simulink model "Hsp"  (Simulink 9.2)
settings: Solver=ode23t  StartTime=0  StopTime=100  FixedStep=0.01  RelTol=1e-3  EnableMultiTasking=on
PreLoadFcn:
  |  Control;HspInit;
values from neighbouring files (symbols this model uses):
  Cep = 1.67    [HspInit.m]    (also in fuzzer_hsp.m; hsp_data.mat)
  Cev = 50.0    (= 50)    [HspInit.m]    (also in fuzzer_hsp.m; hsp_data.mat)
  Cla = 19.23    [HspInit.m]    (also in fuzzer_hsp.m; hsp_data.mat)
  Cpa = 0.76    [HspInit.m]    (also in fuzzer_hsp.m; hsp_data.mat)
  Cpp = 5.80    (= 5.8)    [HspInit.m]    (also in fuzzer_hsp.m; hsp_data.mat)
  Cpv = 25.37    [HspInit.m]    (also in fuzzer_hsp.m; hsp_data.mat)
  Cra = 31.25    [HspInit.m]    (also in fuzzer_hsp.m; hsp_data.mat)
  Csa = 0.28    [HspInit.m]    (also in fuzzer_hsp.m; hsp_data.mat)
  Csp = 2.05    [HspInit.m]    (also in fuzzer_hsp.m; hsp_data.mat)
  Csv = 61.11    [HspInit.m]    (also in fuzzer_hsp.m; hsp_data.mat)
  Dx = [  2     2     2     2    5      5        2   0.2 ]'    [Control.m]    (also in fuzzer_hsp.m; hsp_control.mat = [2 2 2 2 5 5 2 0.2])
  fcs0 = 25    [Control.m]    (also in fuzzer_hsp.m; hsp_control.mat)
  fes0 = 16.11    [Control.m]    (also in fuzzer_hsp.m; hsp_control.mat)
  fes1 = 2.10    (= 2.1)    [Control.m]    (also in fuzzer_hsp.m; hsp_control.mat)
  fesmin = 2.66    [Control.m]    (also in fuzzer_hsp.m; hsp_control.mat)
  fev0 = 3.2    [Control.m]    (also in fuzzer_hsp.m; hsp_control.mat)
  fev1 = 6.3    [Control.m]    (also in fuzzer_hsp.m; hsp_control.mat)
  fmax = 47.78    [Control.m]    (also in fuzzer_hsp.m; hsp_control.mat)
  fmin = 2.52    [Control.m]    (also in fuzzer_hsp.m; hsp_control.mat)
  Gx = [0.475 0.282  0.695 0.53 -265.4 -132.5  -0.13 0.09]'    [Control.m]    (also in fuzzer_hsp.m; hsp_control.mat = [0.475 0.282 0.695 0.53 -265.4 -132.5 -0.13 0.09])
  initx = [2.392 1.412  2.49  0.78 1435.4  1537    0.58   0]'    [Control.m]    (also in fuzzer_hsp.m; hsp_control.mat = [2.392 1.412 2.49 0.78 1435.4 1537 0.58 0])
  ka = 11.758    [Control.m]    (also in fuzzer_hsp.m; hsp_control.mat)
  KElv = 0.014    [HspInit.m]    (also in fuzzer_hsp.m; hsp_data.mat)
  KErv = 0.011    [HspInit.m]    (also in fuzzer_hsp.m; hsp_data.mat)
  kes = 0.0675    [Control.m]    (also in fuzzer_hsp.m; hsp_control.mat)
  kev = 7.06    [Control.m]    (also in fuzzer_hsp.m; hsp_control.mat)
  KRlv = 3.75e-4    (= 0.000375)    [HspInit.m]    (also in fuzzer_hsp.m; hsp_data.mat)
  KRrv = 1.4e-3    (= 0.0014)    [HspInit.m]    (also in fuzzer_hsp.m; hsp_data.mat)
  ksys = 0.075    [HspInit.m]    (also in fuzzer_hsp.m; hsp_data.mat)
  Lpa = 0.18e-3    (= 0.00018)    [HspInit.m]    (also in fuzzer_hsp.m; hsp_data.mat)
  Lsa = 0.22e-3    (= 0.00022)    [HspInit.m]    (also in fuzzer_hsp.m; hsp_data.mat)
  P0lv = 1.5    [HspInit.m]    (also in fuzzer_hsp.m; hsp_data.mat)
  P0rv = 1.5    [HspInit.m]    (also in fuzzer_hsp.m; hsp_data.mat)
  Pn = 92    [Control.m]    (also in fuzzer_hsp.m; hsp_control.mat)
  Rev = 0.016    [HspInit.m]    (also in fuzzer_hsp.m; hsp_data.mat = 0.0336)
  Rla = 25e-3    (= 0.025)    [HspInit.m]    (also in fuzzer_hsp.m; hsp_data.mat)
  Rpa = 0.023    [HspInit.m]    (also in fuzzer_hsp.m; hsp_data.mat = 0.0483)
  Rpp = 0.0894    [HspInit.m]    (also in fuzzer_hsp.m; hsp_data.mat = 0.18774)
  Rpv = 0.0056    [HspInit.m]    (also in fuzzer_hsp.m; hsp_data.mat = 0.01176)
  Rra = 2.5e-3    (= 0.0025)    [HspInit.m]    (also in fuzzer_hsp.m; hsp_data.mat)
  Rsa = 0.06    [HspInit.m]    (also in fuzzer_hsp.m; hsp_data.mat = 0.126)
  Rsv = 0.038    [HspInit.m]    (also in fuzzer_hsp.m; hsp_data.mat = 0.0798)
  toup = 2.076    [Control.m]    (also in fuzzer_hsp.m; hsp_control.mat)
  toux = [  8     8     6     6    20     20       2   1.5 ]'    [Control.m]    (also in fuzzer_hsp.m; hsp_control.mat = [8 8 6 6 20 20 2 1.5])
  touz = 6.37    [Control.m]    (also in fuzzer_hsp.m; hsp_control.mat)
  Tsys0 = 0.5    [HspInit.m]    (also in fuzzer_hsp.m; hsp_data.mat)
  Vt = 5300    [HspInit.m]    (also in fuzzer_hsp.m; hsp_data.mat)
  Vuep = 336.6    [HspInit.m]    (also in fuzzer_hsp.m; hsp_data.mat)
  Vula = 25    [HspInit.m]    (also in fuzzer_hsp.m; hsp_data.mat)
  Vulv = 16.77    [HspInit.m]    (also in fuzzer_hsp.m; hsp_data.mat)
  Vupa = 0    [HspInit.m]    (also in fuzzer_hsp.m; hsp_data.mat)
  Vupp = 123    [HspInit.m]    (also in fuzzer_hsp.m; hsp_data.mat)
  Vupv = 120    [HspInit.m]    (also in fuzzer_hsp.m; hsp_data.mat)
  Vura = 25    [HspInit.m]    (also in fuzzer_hsp.m; hsp_data.mat)
  Vurv = 40.8    [HspInit.m]    (also in fuzzer_hsp.m; hsp_data.mat)
  Vusa = 0    [HspInit.m]    (also in fuzzer_hsp.m; hsp_data.mat)
  Vusp = 274.4    [HspInit.m]    (also in fuzzer_hsp.m; hsp_data.mat)
libraries: simulink x1
CloseFcn:
  | close(findobj(allchild(0),'flat','name','HSP Data Center'));close(findobj(allchild(0),'flat','name','HSP Control Center'))
settings Model: LogicAnalyzerSignalOrdering=c852cb86-1eca-462a-854a-a1c1cbc38954,16da165e-0cbb-4ec2-850a-f71467b3fe42,a6bbb533-7671-4afb-b402-0dcba4b3517f,2284c783-9622-40c3-a6e2-0c1aa7a75d76,7db0d47d-b44d-44ed-95d3-6c2fe47389a0,23f4d4c7-257a-4786-8ae9-d827889f7a35,431a2e10-1d5e-4ec4-bfdf-46f0ec12685f,2c1b38cc-318d-4d33-94a3-ee406883b660,ecc0bcf3-2ebb-404e-884d-df489637ffdc,a0b08e82-c84b-4593-bb1c-8e64f6c8e753,b59d5f8b-8f7e-4c99-855a-97b147fb0b9b,22f6e1f3-01a7-4b2a-becd-6a35e85c0c19,b19c4093-726d-4120-89b8-8ec6b172c3ea,cea4f0ff-484e-4aeb-9f42-7c30204549fe,be0e3e8a-096d-45ad-a129-bf43744257a6  Creator=josie  LastModifiedBy=josie  ExtModeTrigMode=oneshot  ExtModeArmWhenConnect=off
settings Model: LogicAnalyzerGraphicalSettings=|
  | {
  |   "cursors" : {
  |     "activeCursor" : 0,
  |     "lockedCursors" : [
  | 
  |     ],
  |     "startingCursor" : 0,
  |     "times" : [
  |       0
  |     ]
  |   },
  |   "global" : {
  |   },
  |   "panels" : [
  |     {
  |       "height" : 100,
  |       "startingTrace" : 0,
  |       "traces" : [
  |         {
  |           "signalId" : "2284c783-9622-40c3-a6e2-0c1aa7a75d76",
  |           "type" : "wave"
  |         },
  |         {
  |           "signalId" : "2c1b38cc-318d-4d33-94a3-ee406883b660",
  |           "type" : "wave"
  |         },
  |         {
  |           "signalId" : "ecc0bcf3-2ebb-404e-884d-df489637ffdc",
  |           "type" : "wave"
  |         },
  |         {
  |           "signalId" : "a0b08e82-c84b-4593-bb1c-8e64f6c8e753",
  |           "type" : "wave"
  |         },
  |         {
  |           "signalId" : "b59d5f8b-8f7e-4c99-855a-97b147fb0b9b",
  |           "type" : "wave"
  |         },
  |         {
  |           "signalId" : "22f6e1f3-01a7-4b2a-becd-6a35e85c0c19",
  |           "type" : "wave"
  |         },
  |         {
  |           "signalId" : "b19c4093-726d-4120-89b8-8ec6b172c3ea",
  |           "type" : "wave"
  |         },
  |         {
  |           "signalId" : "cea4f0ff-484e-4aeb-9f42-7c30204549fe",
  |           "type" : "wave"
  |         },
  |         {
  |           "signalId" : "be0e3e8a-096d-45ad-a129-bf43744257a6",
  |           "type" : "wave"
  |         },
  |         {
  |           "signalId" : "b284ce3d-31c8-45a4-96bc-bbba7044bc82",
  |           "type" : "wave"
  |         }
  |       ],
  |       "yOffset" : 0
  |     }
  |   ],
  |   "timeAxis" : {
  |     "pixelsPerSecond" : 17.79
  |   },
  |   "trigger" : {
  |     "enabled" : false,
  |     "mode" : "once",
  |     "samples" : 200,
  |     "signals" : {
  |     },
  |     "stages" : [
  |       {
  |         "conditions" : [
  | 
  |         ],
  |         "operator" : "AND"
  |       }
  |     ]
  |   }
  | }
settings DataIOCC: InitialState=xFinal  LimitDataPoints=off  SaveFinalState=on  SignalLoggingSaveFormat=Dataset  SaveOutput=off
settings OptimizationCC: BlockReduction=off  BooleanDataType=off  LifeSpan=auto
settings DebuggingCC: SaveWithParameterizedLinksMsg=none  SignalResolutionControl=TryResolveAllWithWarning  MultiTaskDSMMsg=warning  MultiTaskCondExecSysMsg=none  FcnCallInpInsideContextMsg=error  StateNameClashWarn=none  SFUnexpectedBacktrackingDiag=error  SFNoUnconditionalDefaultTransitionDiag=error  SFExecutionAtInitializationDiag=warning
settings HardwareCC: ProdBitPerPointer=64  ProdBitPerSizeT=64  ProdBitPerPtrDiffT=64  ProdLargestAtomicFloat=Float  ProdIntDivRoundTo=Zero  ProdEndianess=LittleEndian  ProdWordSize=64  ProdHWDeviceType=Intel->x86-64 (Windows64)  TargetUnknown=on
settings SFSimCC: SimUseLocalCustomCode=on
settings RTWCC: RTWUseLocalCustomCode=on
settings CodeAppCC: StateflowObjectComments=off
settings GRTTargetCC: TargetLangStandard=C99 (ISO)  GeneratePreprocessorConditionals=Use local settings
settings ConfigComp: CovMetricSettings=dwe  CovSaveCumulativeToWorkspaceVar=off  CovSaveSingleToWorkspaceVar=off  CovExternalEMLEnable=on

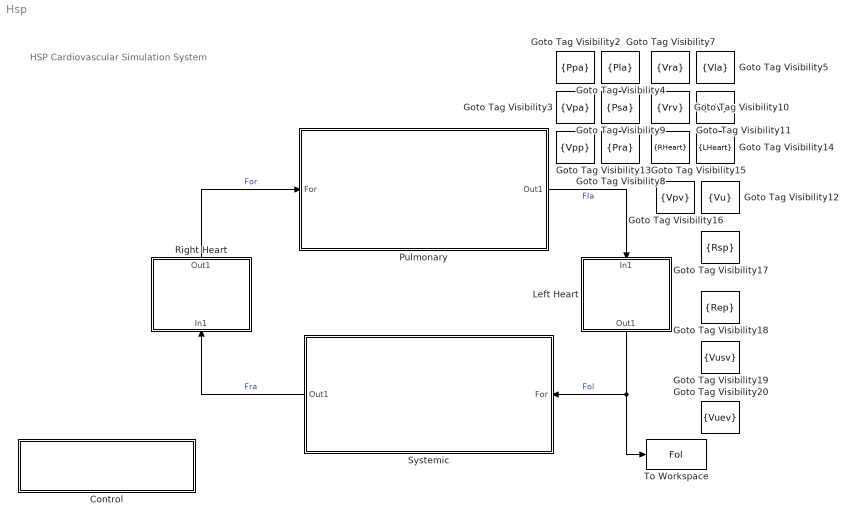
== system Hsp ==
  note: HSP
      | Cardiovascular Simulation System
  Control : Subsystem
      mask Display: disp('ANALYSIS & CONTROL SYSTEM')
  Goto Tag Visibility10 : GotoTagVisibility  GotoTag=Vrv
  Goto Tag Visibility11 : GotoTagVisibility  GotoTag=Vlv
  Goto Tag Visibility12 : GotoTagVisibility  GotoTag=Vu
  Goto Tag Visibility13 : GotoTagVisibility  GotoTag=Vpp
  Goto Tag Visibility14 : GotoTagVisibility  GotoTag=LHeart
  Goto Tag Visibility15 : GotoTagVisibility  GotoTag=RHeart
  Goto Tag Visibility16 : GotoTagVisibility  GotoTag=Vpv
  Goto Tag Visibility17 : GotoTagVisibility  GotoTag=Rsp
  Goto Tag Visibility18 : GotoTagVisibility  GotoTag=Rep
  Goto Tag Visibility19 : GotoTagVisibility  GotoTag=Vusv
  Goto Tag Visibility2 : GotoTagVisibility  GotoTag=Ppa
  Goto Tag Visibility20 : GotoTagVisibility  GotoTag=Vuev
  Goto Tag Visibility3 : GotoTagVisibility  GotoTag=Vpa
  Goto Tag Visibility4 : GotoTagVisibility  GotoTag=Pla
  Goto Tag Visibility5 : GotoTagVisibility  GotoTag=Vla
  Goto Tag Visibility7 : GotoTagVisibility  GotoTag=Vra
  Goto Tag Visibility8 : GotoTagVisibility  GotoTag=Pra
  Goto Tag Visibility9 : GotoTagVisibility  GotoTag=Psa
  Left Heart : Subsystem
      mask Display: disp('LEFT HEART')
  Pulmonary : Subsystem
      mask Display: disp('PULMONARY CIRCULATORY SYSTEM')
  Right Heart : Subsystem
      mask Display: disp('RIGHT HEART')
  Systemic : Subsystem
      mask Display: disp('SYSTEMIC CIRULATORY SYSTEM')
  To Workspace : ToWorkspace  VariableName=Fol  SampleTime=-1
  wires:
  Pulmonary/1(Out1) -> Left Heart/1(In1)  "Fla"
  Systemic/1(Out1) -> Right Heart/1(In1)  "Fra"
  Left Heart/1(Out1) -> Systemic/1(For), To Workspace/1  "Fol"
  Right Heart/1(Out1) -> Pulmonary/1(For)  "For"

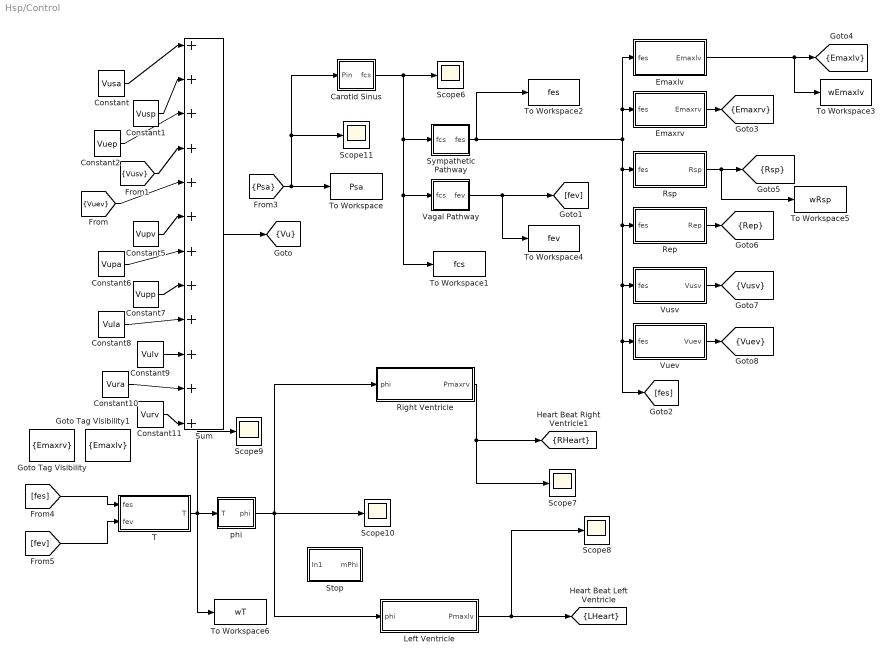
== system Hsp/Control ==
  Carotid Sinus : Subsystem
  Constant : Constant  Value=Vusa
  Constant1 : Constant  Value=Vusp
  Constant10 : Constant  Value=Vura
  Constant11 : Constant  Value=Vurv
  Constant2 : Constant  Value=Vuep
  Constant5 : Constant  Value=Vupv
  Constant6 : Constant  Value=Vupa
  Constant7 : Constant  Value=Vupp
  Constant8 : Constant  Value=Vula
  Constant9 : Constant  Value=Vulv
  Emaxlv : Subsystem
  Emaxrv : Subsystem
  Goto Tag Visibility : GotoTagVisibility  GotoTag=Emaxrv
  Goto Tag Visibility1 : GotoTagVisibility  GotoTag=Emaxlv
  Left Ventricle : Subsystem
  Rep : Subsystem
  Right Ventricle : Subsystem
  Rsp : Subsystem
  Scope{6..11} (6 alike) : Scope
  Stop : Subsystem
  Sum : Sum  Inputs=|++++++++++++  SaturateOnIntegerOverflow=on  InputSameDT=on  OutDataTypeStr=Inherit: Same as first input
  Sympathetic Pathway : Subsystem
  T : Subsystem
  To Workspace : ToWorkspace  VariableName=Psa  SampleTime=-1
  To Workspace1 : ToWorkspace  VariableName=fcs  SampleTime=-1
  To Workspace2 : ToWorkspace  VariableName=fes  SampleTime=-1
  To Workspace3 : ToWorkspace  VariableName=wEmaxlv  SampleTime=-1
  To Workspace4 : ToWorkspace  VariableName=fev  SampleTime=-1
  To Workspace5 : ToWorkspace  VariableName=wRsp  SampleTime=-1
  To Workspace6 : ToWorkspace  VariableName=wT  SampleTime=-1
  Vagal Pathway : Subsystem
  Vuev : Subsystem
  Vusv : Subsystem
  phi : Subsystem
  tag scope: Emaxlv=scoped, Emaxrv=scoped, LHeart=scoped, RHeart=scoped, Rep=scoped, Rsp=scoped, Vu=scoped, Vuev=scoped, Vusv=scoped
  wires:
  Sum/1 -> [Vu]
  Constant/1 -> Sum/1
  Constant2/1 -> Sum/3
  Constant1/1 -> Sum/2
  [Vusv] -> Sum/4
  [Vuev] -> Sum/5
  Constant5/1 -> Sum/6
  Constant6/1 -> Sum/7
  Constant7/1 -> Sum/8
  Constant8/1 -> Sum/9
  Constant9/1 -> Sum/10
  Constant10/1 -> Sum/11
  Constant11/1 -> Sum/12
  Carotid Sinus/1(fcs) -> Scope6/1, Sympathetic Pathway/1(fcs), Vagal Pathway/1(fcs), To Workspace1/1
  [fes] -> T/1(fes)
  [fev] -> T/2(fev)
  phi/1(phi) -> Scope10/1, Right Ventricle/1(phi), Left Ventricle/1(phi)
  Right Ventricle/1(Pmaxrv) -> [RHeart], Scope7/1
  Left Ventricle/1(Pmaxlv) -> [LHeart], Scope8/1
  Sympathetic Pathway/1(fes) -> Emaxlv/1(fes), Emaxrv/1(fes), Rsp/1(fes), Rep/1(fes), Vusv/1(fes), Vuev/1(fes), [fes], To Workspace2/1
  Emaxrv/1(Emaxrv) -> [Emaxrv]
  Rep/1(Rep) -> [Rep]
  Vusv/1(Vusv) -> [Vusv]
  Vuev/1(Vuev) -> [Vuev]
  Vagal Pathway/1(fev) -> [fev], To Workspace4/1
  Rsp/1(Rsp) -> [Rsp], To Workspace5/1
  [Psa] -> To Workspace/1, Scope11/1, Carotid Sinus/1(Pin)
  T/1(T) -> Scope9/1, To Workspace6/1, phi/1(T)
  Emaxlv/1(Emaxlv) -> [Emaxlv], To Workspace3/1

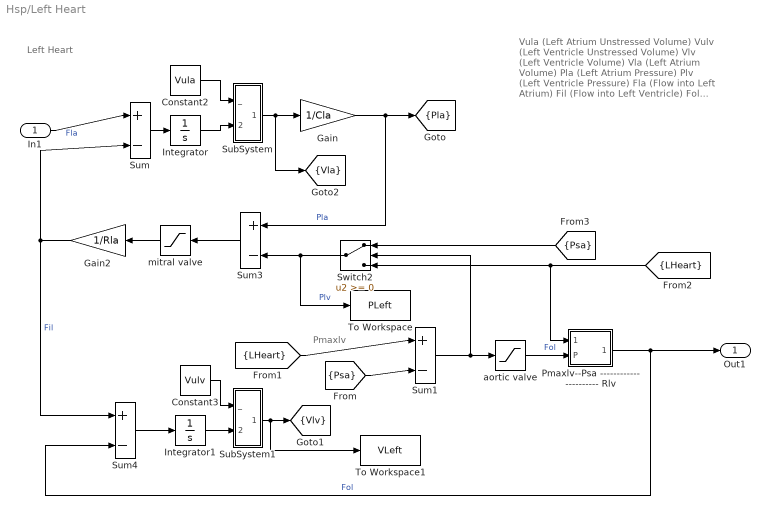
== system Hsp/Left Heart ==
  note: Left Heart
  note: Vula (Left Atrium Unstressed Volume)
      | Vulv (Left Ventricle Unstressed Volume)
      | Vlv (Left Ventricle Volume)
      | Vla (Left Atrium Volume)
      | Pla (Left Atrium Pressure)
      | Plv (Left Ventricle Pressure)
      | Fla (Flow into Left Atrium)
      | Fil (Flow into Left Ventricle)
      | Fol (Flow out of Left Ventricle)
      | LHeart (Left Ventricle Function)
  note: Pmaxlv
  In1 : Inport
  Constant2 : Constant  Value=Vula
  Constant3 : Constant  Value=Vulv
  Gain : Gain  Gain=1/Cla  SaturateOnIntegerOverflow=on  OutDataTypeStr=Inherit: Same as input  ParamDataTypeStr=Inherit: Same as input
  Gain2 : Gain  Gain=1/Rla  SaturateOnIntegerOverflow=on  OutDataTypeStr=Inherit: Same as input  ParamDataTypeStr=Inherit: Same as input
  Integrator : Integrator
  Integrator1 : Integrator
  Pmaxlv--Psa ---------------------- Rlv : Subsystem
  SubSystem : Subsystem
  SubSystem1 : Subsystem
  Sum : Sum  Inputs=|+-  SaturateOnIntegerOverflow=on  InputSameDT=on  OutDataTypeStr=Inherit: Same as first input
  Sum1 : Sum  Inputs=|+-  SaturateOnIntegerOverflow=on  InputSameDT=on  OutDataTypeStr=Inherit: Same as first input
  Sum3 : Sum  Inputs=+-  SaturateOnIntegerOverflow=on  InputSameDT=on  OutDataTypeStr=Inherit: Same as first input
  Sum4 : Sum  Inputs=+-  SaturateOnIntegerOverflow=on  InputSameDT=on  OutDataTypeStr=Inherit: Same as first input
  Switch2 : Switch  SaturateOnIntegerOverflow=on  InputSameDT=on
  To Workspace : ToWorkspace  VariableName=PLeft  SampleTime=-1
  To Workspace1 : ToWorkspace  VariableName=VLeft  SampleTime=-1
  aortic valve : Saturate  UpperLimit=inf  LowerLimit=0
  mitral valve : Saturate  UpperLimit=inf  LowerLimit=0
  Out1 : Outport
  tag scope: Pla=scoped, Vla=scoped, Vlv=scoped
  wires:
  In1/1 -> Sum/1  "Fla"
  Sum/1 -> Integrator/1
  [Psa] -> Sum1/2
  Gain/1 -> [Pla], Sum3/1  "Pla"
  Sum4/1 -> Integrator1/1
  Gain2/1 -> Sum/2, Sum4/1  "Fil"
  Pmaxlv--Psa ---------------------- Rlv/1(Flow) -> Out1/1, Sum4/2  "Fol"
  Constant2/1 -> SubSystem/1(_)
  Constant3/1 -> SubSystem1/1(_)
  SubSystem/1(Out) -> Gain/1, [Vla]
  [LHeart] -> Sum1/1
  Sum1/1 -> aortic valve/1, Switch2/2
  [Psa] -> Switch2/1
  mitral valve/1 -> Gain2/1
  [LHeart] -> Switch2/3, Pmaxlv--Psa ---------------------- Rlv/1(Pmax)
  aortic valve/1 -> Pmaxlv--Psa ---------------------- Rlv/2(P)  "Fol"
  Switch2/1 -> Sum3/2, To Workspace/1  "Plv"
  SubSystem1/1(Out) -> [Vlv], To Workspace1/1
  Integrator1/1 -> SubSystem1/2(+)
  Sum3/1 -> mitral valve/1
  Integrator/1 -> SubSystem/2(+)

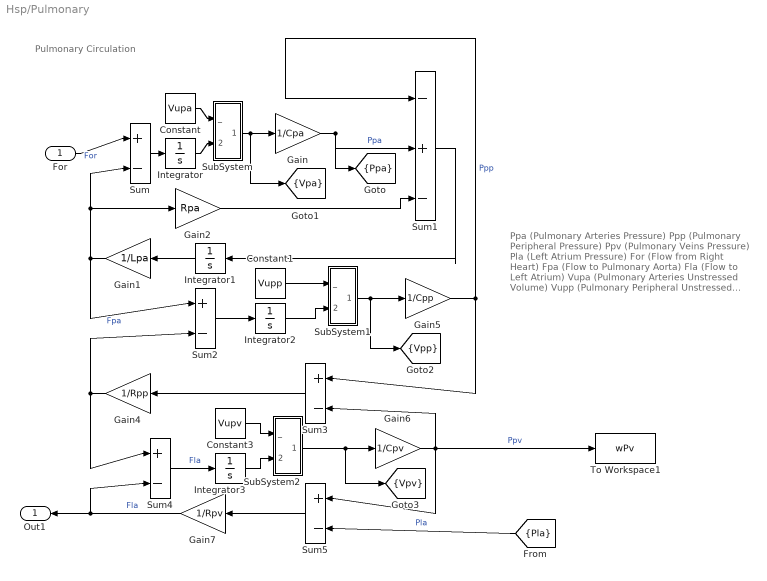
== system Hsp/Pulmonary ==
  note: Ppa (Pulmonary Arteries Pressure)
      | Ppp (Pulmonary Peripheral Pressure)
      | Ppv (Pulmonary Veins Pressure)
      | Pla (Left Atrium Pressure)
      | For (Flow from Right Heart)
      | Fpa (Flow to Pulmonary Aorta)
      | Fla (Flow to Left Atrium)
      | Vupa (Pulmonary Arteries Unstressed Volume)
      | Vupp (Pulmonary Peripheral Unstressed Volume)
      | Vupv (Pulmonary Veins Unstressed Volume)
  note: Pulmonary Circulation
  For : Inport
  Constant : Constant  Value=Vupa
  Constant1 : Constant  Value=Vupp
  Constant3 : Constant  Value=Vupv
  Gain : Gain  Gain=1/Cpa  SaturateOnIntegerOverflow=on  OutDataTypeStr=Inherit: Same as input  ParamDataTypeStr=Inherit: Same as input
  Gain1 : Gain  Gain=1/Lpa  SaturateOnIntegerOverflow=on  OutDataTypeStr=Inherit: Same as input  ParamDataTypeStr=Inherit: Same as input
  Gain2 : Gain  Gain=Rpa  SaturateOnIntegerOverflow=on  OutDataTypeStr=Inherit: Same as input  ParamDataTypeStr=Inherit: Same as input
  Gain4 : Gain  Gain=1/Rpp  SaturateOnIntegerOverflow=on  OutDataTypeStr=Inherit: Same as input  ParamDataTypeStr=Inherit: Same as input
  Gain5 : Gain  Gain=1/Cpp  SaturateOnIntegerOverflow=on  OutDataTypeStr=Inherit: Same as input  ParamDataTypeStr=Inherit: Same as input
  Gain6 : Gain  Gain=1/Cpv  SaturateOnIntegerOverflow=on  OutDataTypeStr=Inherit: Same as input  ParamDataTypeStr=Inherit: Same as input
  Gain7 : Gain  Gain=1/Rpv  SaturateOnIntegerOverflow=on  OutDataTypeStr=Inherit: Same as input  ParamDataTypeStr=Inherit: Same as input
  Integrator : Integrator  InitialCondition=100
  Integrator1 : Integrator
  Integrator2 : Integrator  InitialCondition=100
  Integrator3 : Integrator
  SubSystem : Subsystem
  SubSystem1 : Subsystem
  SubSystem2 : Subsystem
  Sum{,2..5} (5 alike) : Sum  Inputs=|+-  SaturateOnIntegerOverflow=on  InputSameDT=on  OutDataTypeStr=Inherit: Same as first input
  Sum1 : Sum  Inputs=|-+-  SaturateOnIntegerOverflow=on  InputSameDT=on  OutDataTypeStr=Inherit: Same as first input
  To Workspace1 : ToWorkspace  VariableName=wPv  SampleTime=-1
  Out1 : Outport
  tag scope: Ppa=scoped, Vpa=scoped, Vpp=scoped, Vpv=scoped
  wires:
  For/1 -> Sum/1  "For"
  Sum/1 -> Integrator/1
  Integrator1/1 -> Gain1/1
  Sum1/1 -> Integrator1/1
  Gain2/1 -> Sum1/3
  Gain1/1 -> Sum/2, Gain2/1, Sum2/1  "Fpa"
  Sum2/1 -> Integrator2/1
  Gain5/1 -> Sum1/1, Sum3/1  "Ppp"
  Sum3/1 -> Gain4/1
  Gain4/1 -> Sum2/2, Sum4/1
  Sum5/1 -> Gain7/1
  Gain6/1 -> Sum3/2, Sum5/1, To Workspace1/1  "Ppv"
  [Pla] -> Sum5/2  "Pla"
  Sum4/1 -> Integrator3/1  "Fla"
  Gain/1 -> Sum1/2, [Ppa]  "Ppa"
  SubSystem/1(Out) -> Gain/1, [Vpa]
  SubSystem1/1(Out) -> Gain5/1, [Vpp]
  SubSystem2/1(Out) -> Gain6/1, [Vpv]
  Integrator/1 -> SubSystem/2(+)
  Constant/1 -> SubSystem/1(_)
  Constant1/1 -> SubSystem1/1(_)
  Integrator2/1 -> SubSystem1/2(+)
  Integrator3/1 -> SubSystem2/2(+)
  Gain7/1 -> Sum4/2, Out1/1  "Fla"
  Constant3/1 -> SubSystem2/1(_)

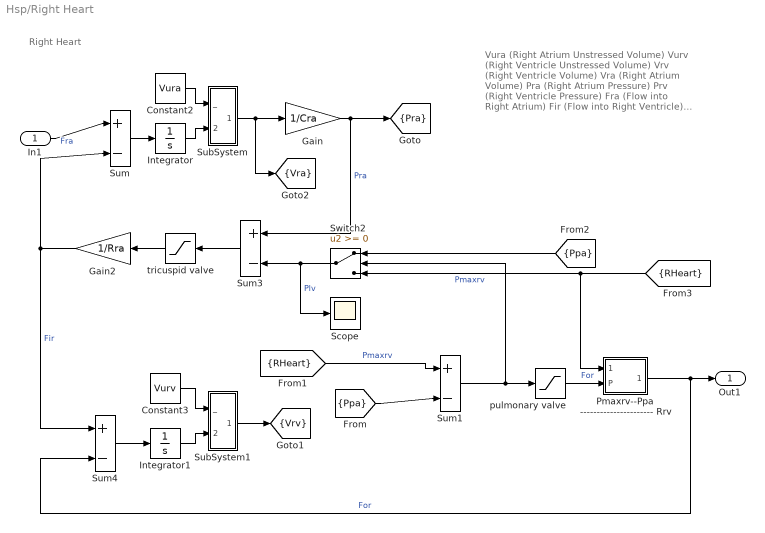
== system Hsp/Right Heart ==
  note: Right Heart
  note: Vura (Right Atrium Unstressed Volume)
      | Vurv (Right Ventricle Unstressed Volume)
      | Vrv (Right Ventricle Volume)
      | Vra (Right Atrium Volume)
      | Pra (Right Atrium Pressure)
      | Prv (Right Ventricle Pressure)
      | Fra (Flow into Right Atrium)
      | Fir (Flow into Right Ventricle)
      | For (Flow out of Right Ventricle)
      | LHeart (Left Ventricle Function)
  In1 : Inport
  Constant2 : Constant  Value=Vura
  Constant3 : Constant  Value=Vurv
  Gain : Gain  Gain=1/Cra  SaturateOnIntegerOverflow=on  OutDataTypeStr=Inherit: Same as input  ParamDataTypeStr=Inherit: Same as input
  Gain2 : Gain  Gain=1/Rra  SaturateOnIntegerOverflow=on  OutDataTypeStr=Inherit: Same as input  ParamDataTypeStr=Inherit: Same as input
  Integrator : Integrator
  Integrator1 : Integrator
  Pmaxrv--Ppa ---------------------- Rrv : Subsystem
  Scope : Scope
  SubSystem : Subsystem
  SubSystem1 : Subsystem
  Sum : Sum  Inputs=|+-  SaturateOnIntegerOverflow=on  InputSameDT=on  OutDataTypeStr=Inherit: Same as first input
  Sum1 : Sum  Inputs=|+-  SaturateOnIntegerOverflow=on  InputSameDT=on  OutDataTypeStr=Inherit: Same as first input
  Sum3 : Sum  Inputs=+-  SaturateOnIntegerOverflow=on  InputSameDT=on  OutDataTypeStr=Inherit: Same as first input
  Sum4 : Sum  Inputs=+-  SaturateOnIntegerOverflow=on  InputSameDT=on  OutDataTypeStr=Inherit: Same as first input
  Switch2 : Switch  SaturateOnIntegerOverflow=on  InputSameDT=on
  pulmonary valve : Saturate  UpperLimit=inf  LowerLimit=0
  tricuspid valve : Saturate  UpperLimit=inf  LowerLimit=0
  Out1 : Outport
  tag scope: Pra=scoped, Vra=scoped, Vrv=scoped
  wires:
  In1/1 -> Sum/1  "Fra"
  Sum/1 -> Integrator/1
  [Ppa] -> Sum1/2
  Gain/1 -> [Pra], Sum3/1  "Pra"
  Gain2/1 -> Sum/2, Sum4/1  "Fir"
  Integrator/1 -> SubSystem/2(+)
  Constant2/1 -> SubSystem/1(_)
  SubSystem1/1(Out) -> [Vrv]
  SubSystem/1(Out) -> Gain/1, [Vra]
  Constant3/1 -> SubSystem1/1(_)
  Integrator1/1 -> SubSystem1/2(+)
  [RHeart] -> Sum1/1  "Pmaxrv"
  Sum1/1 -> pulmonary valve/1, Switch2/2
  [Ppa] -> Switch2/1
  tricuspid valve/1 -> Gain2/1
  pulmonary valve/1 -> Pmaxrv--Ppa ---------------------- Rrv/2(P)  "For"
  Pmaxrv--Ppa ---------------------- Rrv/1(Flow) -> Out1/1, Sum4/2  "For"
  [RHeart] -> Switch2/3, Pmaxrv--Ppa ---------------------- Rrv/1(Pmax)  "Pmaxrv"
  Sum4/1 -> Integrator1/1
  Sum3/1 -> tricuspid valve/1
  Switch2/1 -> Sum3/2, Scope/1  "Plv"

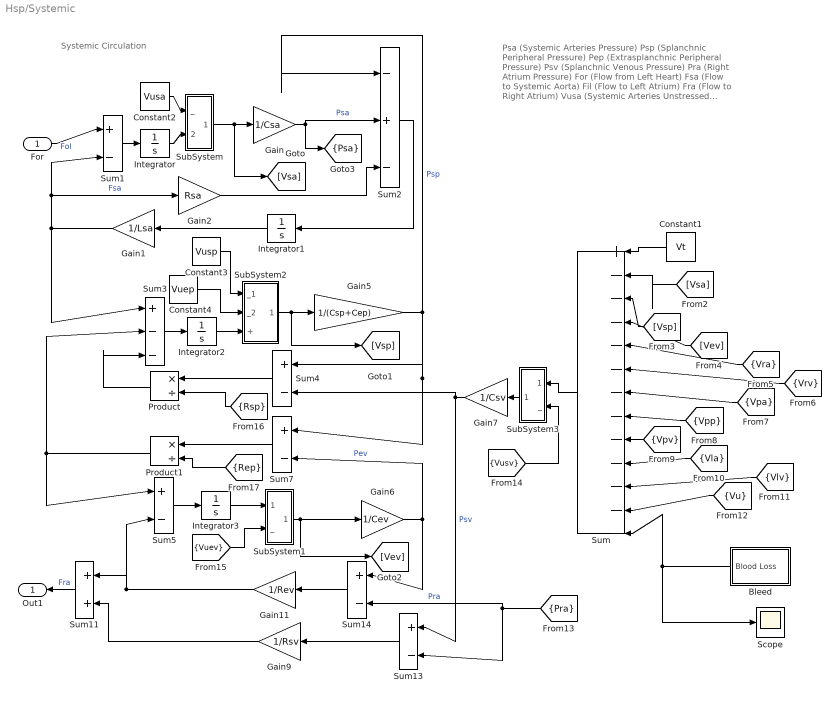
== system Hsp/Systemic ==
  note: Psa (Systemic Arteries Pressure)
      | Psp (Splanchnic Peripheral Pressure)
      | Pep (Extrasplanchnic Peripheral Pressure)
      | Psv (Splanchnic Venous Pressure)
      | Pra (Right Atrium Pressure)
      | For (Flow from Left Heart)
      | Fsa (Flow to Systemic Aorta)
      | Fil (Flow to Left Atrium)
      | Fra (Flow to Right Atrium)
      | Vusa (Systemic Arteries Unstressed Volume)
      | Vusp (Extrasplanchnic Venous Unstressed Volume)
      | Vuep (Splanchnic Venous Unstressed Volume)
      | Vuev (Extrasplanchnic Venous Unstressed Volume)
      | Vusv (Splanchnic Venous Unstressed Volume)
  note: Systemic Circulation
  For : Inport
  Bleed : Subsystem  mask{ulimit=0, rate=0, tstart=0}
      mask prompts: ulimit "Bleed Up Limit (ml)"; rate "Bleed Rate (ml/s)"; tstart "Bleed Start Time (s)"
  Constant1 : Constant  Value=Vt
  Constant2 : Constant  Value=Vusa
  Constant3 : Constant  Value=Vusp
  Constant4 : Constant  Value=Vuep
  Gain : Gain  Gain=1/Csa  SaturateOnIntegerOverflow=on  OutDataTypeStr=Inherit: Same as input  ParamDataTypeStr=Inherit: Same as input
  Gain1 : Gain  Gain=1/Lsa  SaturateOnIntegerOverflow=on  OutDataTypeStr=Inherit: Same as input  ParamDataTypeStr=Inherit: Same as input
  Gain11 : Gain  Gain=1/Rev  SaturateOnIntegerOverflow=on  OutDataTypeStr=Inherit: Same as input  ParamDataTypeStr=Inherit: Same as input
  Gain2 : Gain  Gain=Rsa  SaturateOnIntegerOverflow=on  OutDataTypeStr=Inherit: Same as input  ParamDataTypeStr=Inherit: Same as input
  Gain5 : Gain  Gain=1/(Csp+Cep)  SaturateOnIntegerOverflow=on  OutDataTypeStr=Inherit: Same as input  ParamDataTypeStr=Inherit: Same as input
  Gain6 : Gain  Gain=1/Cev  SaturateOnIntegerOverflow=on  OutDataTypeStr=Inherit: Same as input  ParamDataTypeStr=Inherit: Same as input
  Gain7 : Gain  Gain=1/Csv  SaturateOnIntegerOverflow=on  OutDataTypeStr=Inherit: Same as input  ParamDataTypeStr=Inherit: Same as input
  Gain9 : Gain  Gain=1/Rsv  SaturateOnIntegerOverflow=on  OutDataTypeStr=Inherit: Same as input  ParamDataTypeStr=Inherit: Same as input
  Integrator{,1..3} (4 alike) : Integrator
  Product : Product  Inputs=*/  SaturateOnIntegerOverflow=on  RndMeth=Zero  InputSameDT=on  OutDataTypeStr=Inherit: Same as first input
  Product1 : Product  Inputs=*/  SaturateOnIntegerOverflow=on  RndMeth=Zero  InputSameDT=on  OutDataTypeStr=Inherit: Same as first input
  Scope : Scope
  SubSystem : Subsystem
  SubSystem1 : Subsystem
  SubSystem2 : Subsystem
  SubSystem3 : Subsystem
  Sum : Sum  Inputs=|+------------  SaturateOnIntegerOverflow=on  InputSameDT=on  OutDataTypeStr=Inherit: Same as first input
  Sum{1,4..5,7,13..14} (6 alike) : Sum  Inputs=|+-  SaturateOnIntegerOverflow=on  InputSameDT=on  OutDataTypeStr=Inherit: Same as first input
  Sum11 : Sum  Inputs=|++  SaturateOnIntegerOverflow=on  InputSameDT=on  OutDataTypeStr=Inherit: Same as first input
  Sum2 : Sum  Inputs=|-+-  SaturateOnIntegerOverflow=on  InputSameDT=on  OutDataTypeStr=Inherit: Same as first input
  Sum3 : Sum  Inputs=|+--  SaturateOnIntegerOverflow=on  InputSameDT=on  OutDataTypeStr=Inherit: Same as first input
  Out1 : Outport
  tag scope: Psa=scoped
  wires:
  For/1 -> Sum1/1  "Fol"
  Sum1/1 -> Integrator/1
  Integrator1/1 -> Gain1/1
  Sum2/1 -> Integrator1/1
  Gain2/1 -> Sum2/3
  Gain1/1 -> Sum1/2, Gain2/1, Sum3/1  "Fsa"
  Sum3/1 -> Integrator2/1
  Gain5/1 -> Sum2/1, Sum4/1, Sum7/1  "Psp"
  Product/1 -> Sum3/3
  Product1/1 -> Sum3/2, Sum5/1
  Integrator3/1 -> SubSystem1/1(+)
  SubSystem1/1(Out) -> Gain6/1, [Vev]
  Constant1/1 -> Sum/1
  [Vsa] -> Sum/2
  [Vsp] -> Sum/3
  [Vev] -> Sum/4
  [Vra] -> Sum/5
  [Vrv] -> Sum/6
  [Vpa] -> Sum/7
  [Vpp] -> Sum/8
  [Vpv] -> Sum/9
  [Vla] -> Sum/10
  [Vlv] -> Sum/11
  [Vu] -> Sum/12
  Integrator/1 -> SubSystem/2(+)
  SubSystem/1(Out) -> Gain/1, [Vsa]
  Integrator2/1 -> SubSystem2/3(+)
  SubSystem2/1(Out) -> Gain5/1, [Vsp]
  SubSystem3/1(Out) -> Gain7/1
  Sum13/1 -> Gain9/1
  Sum11/1 -> Out1/1  "Fra"
  Gain7/1 -> Sum4/2, Sum13/1  "Psv"
  Gain9/1 -> Sum11/2
  Gain6/1 -> Sum7/2, Sum14/1  "Pev"
  Sum14/1 -> Gain11/1
  [Pra] -> Sum13/2, Sum14/2  "Pra"
  Sum5/1 -> Integrator3/1
  Gain11/1 -> Sum11/1, Sum5/2
  Gain/1 -> Sum2/2, [Psa]  "Psa"
  Constant2/1 -> SubSystem/1(_)
  [Vuev] -> SubSystem1/2(_)
  Constant3/1 -> SubSystem2/1(_1)
  Constant4/1 -> SubSystem2/2(_2)
  Sum/1 -> SubSystem3/1(+)
  [Vusv] -> SubSystem3/2(_)
  Sum4/1 -> Product/1
  [Rsp] -> Product/2
  [Rep] -> Product1/2
  Sum7/1 -> Product1/1
  Bleed/1(Blood Loss) -> Sum/13, Scope/1

== system Hsp/Control/Carotid Sinus ==
  Pin : Inport
  Fcn : Fcn  Expr=(fmin+fmax*exp((u-Pn)/ka))/(1+exp((u-Pn)/ka))
  Transfer Fcn : TransferFcn  Numerator=[touz 1]  Denominator=[toup 1]
  fcs : Outport
  wires:
  Pin/1 -> Transfer Fcn/1
  Transfer Fcn/1 -> Fcn/1
  Fcn/1 -> fcs/1

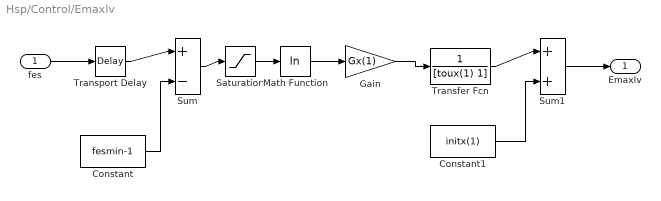
== system Hsp/Control/Emaxlv ==
  fes : Inport
  Constant : Constant  Value=fesmin-1
  Constant1 : Constant  Value=initx(1)
  Gain : Gain  Gain=Gx(1)  SaturateOnIntegerOverflow=on  OutDataTypeStr=Inherit: Same as input  ParamDataTypeStr=Inherit: Same as input
  Math Function : Math  Operator=log  SaturateOnIntegerOverflow=on
  Saturation : Saturate  UpperLimit=inf  LowerLimit=1
  Sum : Sum  Inputs=|+-  SaturateOnIntegerOverflow=on  InputSameDT=on  OutDataTypeStr=Inherit: Same as first input
  Sum1 : Sum  Inputs=|++  SaturateOnIntegerOverflow=on  InputSameDT=on  OutDataTypeStr=Inherit: Same as first input
  Transfer Fcn : TransferFcn  Denominator=[toux(1) 1]
  Transport Delay : TransportDelay  DelayTime=Dx(1)
  Emaxlv : Outport
  wires:
  fes/1 -> Transport Delay/1
  Transport Delay/1 -> Sum/1
  Constant/1 -> Sum/2
  Sum/1 -> Saturation/1
  Saturation/1 -> Math Function/1
  Math Function/1 -> Gain/1
  Gain/1 -> Transfer Fcn/1
  Transfer Fcn/1 -> Sum1/1
  Sum1/1 -> Emaxlv/1
  Constant1/1 -> Sum1/2

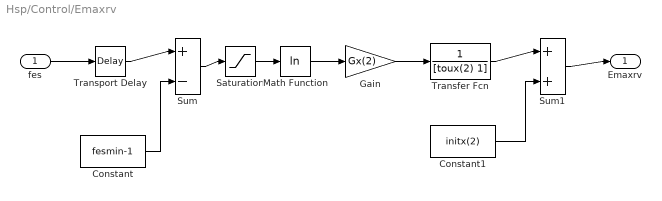
== system Hsp/Control/Emaxrv ==
  fes : Inport
  Constant : Constant  Value=fesmin-1
  Constant1 : Constant  Value=initx(2)
  Gain : Gain  Gain=Gx(2)  SaturateOnIntegerOverflow=on  OutDataTypeStr=Inherit: Same as input  ParamDataTypeStr=Inherit: Same as input
  Math Function : Math  Operator=log  SaturateOnIntegerOverflow=on
  Saturation : Saturate  UpperLimit=inf  LowerLimit=1
  Sum : Sum  Inputs=|+-  SaturateOnIntegerOverflow=on  InputSameDT=on  OutDataTypeStr=Inherit: Same as first input
  Sum1 : Sum  Inputs=|++  SaturateOnIntegerOverflow=on  InputSameDT=on  OutDataTypeStr=Inherit: Same as first input
  Transfer Fcn : TransferFcn  Denominator=[toux(2) 1]
  Transport Delay : TransportDelay  DelayTime=Dx(2)
  Emaxrv : Outport
  wires:
  Constant1/1 -> Sum1/2
  Sum1/1 -> Emaxrv/1
  Transfer Fcn/1 -> Sum1/1
  Gain/1 -> Transfer Fcn/1
  Math Function/1 -> Gain/1
  Saturation/1 -> Math Function/1
  Sum/1 -> Saturation/1
  Constant/1 -> Sum/2
  Transport Delay/1 -> Sum/1
  fes/1 -> Transport Delay/1

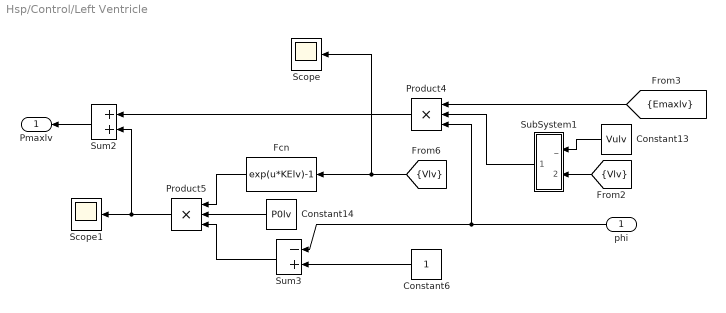
== system Hsp/Control/Left Ventricle ==
  phi : Inport
  Constant13 : Constant  Value=Vulv
  Constant14 : Constant  Value=P0lv
  Constant6 : Constant
  Fcn : Fcn  Expr=exp(u*KElv)-1
  Product4 : Product  Inputs=3  SaturateOnIntegerOverflow=on  RndMeth=Zero  InputSameDT=on  OutDataTypeStr=Inherit: Same as first input
  Product5 : Product  Inputs=3  SaturateOnIntegerOverflow=on  RndMeth=Zero  InputSameDT=on  OutDataTypeStr=Inherit: Same as first input
  Scope : Scope
  Scope1 : Scope
  SubSystem1 : Subsystem
  Sum2 : Sum  SaturateOnIntegerOverflow=on  InputSameDT=on  OutDataTypeStr=Inherit: Same as first input
  Sum3 : Sum  Inputs=-+  SaturateOnIntegerOverflow=on  InputSameDT=on  OutDataTypeStr=Inherit: Same as first input
  Pmaxlv : Outport
  wires:
  Sum2/1 -> Pmaxlv/1
  Product4/1 -> Sum2/1
  Product5/1 -> Sum2/2, Scope1/1
  Fcn/1 -> Product5/1
  Constant14/1 -> Product5/2
  Sum3/1 -> Product5/3
  Constant6/1 -> Sum3/2
  Constant13/1 -> SubSystem1/1(_)
  [Vlv] -> SubSystem1/2(+)
  SubSystem1/1(Out) -> Product4/2
  phi/1 -> Sum3/1, Product4/3
  [Emaxlv] -> Product4/1
  [Vlv] -> Fcn/1, Scope/1

== system Hsp/Control/Rep ==
  fes : Inport
  Constant : Constant  Value=fesmin-1
  Constant1 : Constant  Value=initx(4)
  Gain : Gain  Gain=Gx(4)  SaturateOnIntegerOverflow=on  OutDataTypeStr=Inherit: Same as input  ParamDataTypeStr=Inherit: Same as input
  Math Function : Math  Operator=log  SaturateOnIntegerOverflow=on
  Saturation : Saturate  UpperLimit=inf  LowerLimit=1
  Sum : Sum  Inputs=|+-  SaturateOnIntegerOverflow=on  InputSameDT=on  OutDataTypeStr=Inherit: Same as first input
  Sum1 : Sum  Inputs=|++  SaturateOnIntegerOverflow=on  InputSameDT=on  OutDataTypeStr=Inherit: Same as first input
  Transfer Fcn : TransferFcn  Denominator=[toux(4) 1]
  Transport Delay : TransportDelay  DelayTime=Dx(4)
  Rep : Outport
  wires:
  Constant1/1 -> Sum1/2
  Sum1/1 -> Rep/1
  Transfer Fcn/1 -> Sum1/1
  Gain/1 -> Transfer Fcn/1
  Math Function/1 -> Gain/1
  Saturation/1 -> Math Function/1
  Sum/1 -> Saturation/1
  Constant/1 -> Sum/2
  Transport Delay/1 -> Sum/1
  fes/1 -> Transport Delay/1

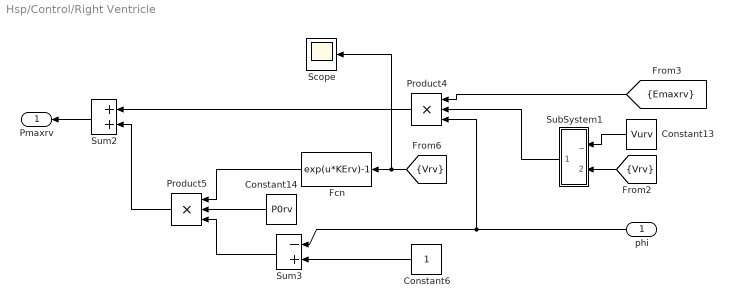
== system Hsp/Control/Right Ventricle ==
  phi : Inport
  Constant13 : Constant  Value=Vurv
  Constant14 : Constant  Value=P0rv
  Constant6 : Constant
  Fcn : Fcn  Expr=exp(u*KErv)-1
  Product4 : Product  Inputs=3  SaturateOnIntegerOverflow=on  RndMeth=Zero  InputSameDT=on  OutDataTypeStr=Inherit: Same as first input
  Product5 : Product  Inputs=3  SaturateOnIntegerOverflow=on  RndMeth=Zero  InputSameDT=on  OutDataTypeStr=Inherit: Same as first input
  Scope : Scope
  SubSystem1 : Subsystem
  Sum2 : Sum  SaturateOnIntegerOverflow=on  InputSameDT=on  OutDataTypeStr=Inherit: Same as first input
  Sum3 : Sum  Inputs=-+  SaturateOnIntegerOverflow=on  InputSameDT=on  OutDataTypeStr=Inherit: Same as first input
  Pmaxrv : Outport
  wires:
  Constant6/1 -> Sum3/2
  Sum3/1 -> Product5/3
  Constant14/1 -> Product5/2
  Fcn/1 -> Product5/1
  Product5/1 -> Sum2/2
  Product4/1 -> Sum2/1
  Sum2/1 -> Pmaxrv/1
  [Emaxrv] -> Product4/1
  [Vrv] -> SubSystem1/2(+)
  Constant13/1 -> SubSystem1/1(_)
  SubSystem1/1(Out) -> Product4/2
  phi/1 -> Sum3/1, Product4/3
  [Vrv] -> Fcn/1, Scope/1

== system Hsp/Control/Rsp ==
  fes : Inport
  Constant : Constant  Value=fesmin-1
  Constant1 : Constant  Value=initx(3)
  Gain : Gain  Gain=Gx(3)  SaturateOnIntegerOverflow=on  OutDataTypeStr=Inherit: Same as input  ParamDataTypeStr=Inherit: Same as input
  Math Function : Math  Operator=log  SaturateOnIntegerOverflow=on
  Saturation : Saturate  UpperLimit=inf  LowerLimit=1
  Sum : Sum  Inputs=|+-  SaturateOnIntegerOverflow=on  InputSameDT=on  OutDataTypeStr=Inherit: Same as first input
  Sum1 : Sum  Inputs=|++  SaturateOnIntegerOverflow=on  InputSameDT=on  OutDataTypeStr=Inherit: Same as first input
  Transfer Fcn : TransferFcn  Denominator=[toux(3) 1]
  Transport Delay : TransportDelay  DelayTime=Dx(3)
  Rsp : Outport
  wires:
  fes/1 -> Transport Delay/1
  Transport Delay/1 -> Sum/1
  Constant/1 -> Sum/2
  Sum/1 -> Saturation/1
  Saturation/1 -> Math Function/1
  Math Function/1 -> Gain/1
  Gain/1 -> Transfer Fcn/1
  Transfer Fcn/1 -> Sum1/1
  Sum1/1 -> Rsp/1
  Constant1/1 -> Sum1/2

== system Hsp/Control/Stop ==
  In1 : Inport
  Clock : Clock
  Constant : Constant  Value=0
  Switch : Switch  Threshold=50  SaturateOnIntegerOverflow=on  InputSameDT=on
  mPhi : Outport
  wires:
  In1/1 -> Switch/3
  Constant/1 -> Switch/1
  Switch/1 -> mPhi/1
  Clock/1 -> Switch/2

== system Hsp/Control/Sympathetic Pathway ==
  fcs : Inport
  Constant : Constant  Value=fes1
  Gain : Gain  Gain=-kes  SaturateOnIntegerOverflow=on  OutDataTypeStr=Inherit: Same as input  ParamDataTypeStr=Inherit: Same as input
  Gain1 : Gain  Gain=fes0-fes1  SaturateOnIntegerOverflow=on  OutDataTypeStr=Inherit: Same as input  ParamDataTypeStr=Inherit: Same as input
  Math Function : Math  SaturateOnIntegerOverflow=on
  Sum : Sum  Inputs=|++  SaturateOnIntegerOverflow=on  InputSameDT=on  OutDataTypeStr=Inherit: Same as first input
  fes : Outport
  wires:
  Gain1/1 -> Sum/1
  Constant/1 -> Sum/2
  Sum/1 -> fes/1
  fcs/1 -> Gain/1
  Gain/1 -> Math Function/1
  Math Function/1 -> Gain1/1

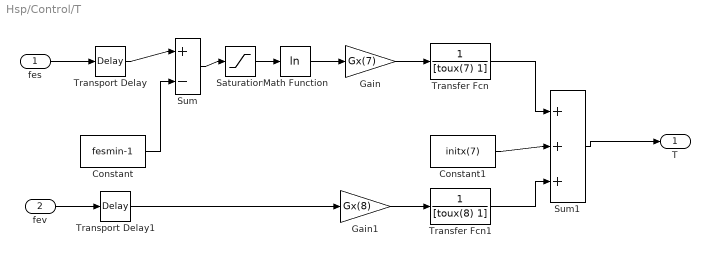
== system Hsp/Control/T ==
  fes : Inport
  fev : Inport  Port=2
  Constant : Constant  Value=fesmin-1
  Constant1 : Constant  Value=initx(7)
  Gain : Gain  Gain=Gx(7)  SaturateOnIntegerOverflow=on  OutDataTypeStr=Inherit: Same as input  ParamDataTypeStr=Inherit: Same as input
  Gain1 : Gain  Gain=Gx(8)  SaturateOnIntegerOverflow=on  OutDataTypeStr=Inherit: Same as input  ParamDataTypeStr=Inherit: Same as input
  Math Function : Math  Operator=log  SaturateOnIntegerOverflow=on
  Saturation : Saturate  UpperLimit=inf  LowerLimit=1
  Sum : Sum  Inputs=|+-  SaturateOnIntegerOverflow=on  InputSameDT=on  OutDataTypeStr=Inherit: Same as first input
  Sum1 : Sum  Inputs=|+++  SaturateOnIntegerOverflow=on  InputSameDT=on  OutDataTypeStr=Inherit: Same as first input
  Transfer Fcn : TransferFcn  Denominator=[toux(7) 1]
  Transfer Fcn1 : TransferFcn  Denominator=[toux(8) 1]
  Transport Delay : TransportDelay  DelayTime=Dx(7)
  Transport Delay1 : TransportDelay  DelayTime=Dx(8)
  T : Outport
  wires:
  fes/1 -> Transport Delay/1
  Transport Delay/1 -> Sum/1
  Constant/1 -> Sum/2
  Sum/1 -> Saturation/1
  Saturation/1 -> Math Function/1
  Math Function/1 -> Gain/1
  Gain/1 -> Transfer Fcn/1
  Transfer Fcn/1 -> Sum1/1
  Sum1/1 -> T/1
  Constant1/1 -> Sum1/2
  fev/1 -> Transport Delay1/1
  Transport Delay1/1 -> Gain1/1
  Gain1/1 -> Transfer Fcn1/1
  Transfer Fcn1/1 -> Sum1/3

== system Hsp/Control/Vagal Pathway ==
  fcs : Inport
  Fcn : Fcn  Expr=(fev0+fev1*exp((u-fcs0)/kev))/(1+exp((u-fcs0)/kev))
  fev : Outport
  wires:
  Fcn/1 -> fev/1
  fcs/1 -> Fcn/1

== system Hsp/Control/Vuev ==
  fes : Inport
  Constant : Constant  Value=fesmin-1
  Constant1 : Constant  Value=initx(6)
  Gain : Gain  Gain=Gx(6)  SaturateOnIntegerOverflow=on  OutDataTypeStr=Inherit: Same as input  ParamDataTypeStr=Inherit: Same as input
  Math Function : Math  Operator=log  SaturateOnIntegerOverflow=on
  Saturation : Saturate  UpperLimit=inf  LowerLimit=1
  Sum : Sum  Inputs=|+-  SaturateOnIntegerOverflow=on  InputSameDT=on  OutDataTypeStr=Inherit: Same as first input
  Sum1 : Sum  Inputs=|++  SaturateOnIntegerOverflow=on  InputSameDT=on  OutDataTypeStr=Inherit: Same as first input
  Transfer Fcn : TransferFcn  Denominator=[toux(6) 1]
  Transport Delay : TransportDelay  DelayTime=Dx(6)
  Vuev : Outport
  wires:
  Constant1/1 -> Sum1/2
  Sum1/1 -> Vuev/1
  Transfer Fcn/1 -> Sum1/1
  Gain/1 -> Transfer Fcn/1
  Math Function/1 -> Gain/1
  Saturation/1 -> Math Function/1
  Sum/1 -> Saturation/1
  Constant/1 -> Sum/2
  Transport Delay/1 -> Sum/1
  fes/1 -> Transport Delay/1

== system Hsp/Control/Vusv ==
  fes : Inport
  Constant : Constant  Value=fesmin-1
  Constant1 : Constant  Value=initx(5)
  Gain : Gain  Gain=Gx(5)  SaturateOnIntegerOverflow=on  OutDataTypeStr=Inherit: Same as input  ParamDataTypeStr=Inherit: Same as input
  Math Function : Math  Operator=log  SaturateOnIntegerOverflow=on
  Saturation : Saturate  UpperLimit=inf  LowerLimit=1
  Sum : Sum  Inputs=|+-  SaturateOnIntegerOverflow=on  InputSameDT=on  OutDataTypeStr=Inherit: Same as first input
  Sum1 : Sum  Inputs=|++  SaturateOnIntegerOverflow=on  InputSameDT=on  OutDataTypeStr=Inherit: Same as first input
  Transfer Fcn : TransferFcn  Denominator=[toux(5) 1]
  Transport Delay : TransportDelay  DelayTime=Dx(5)
  Vusv : Outport
  wires:
  fes/1 -> Transport Delay/1
  Transport Delay/1 -> Sum/1
  Constant/1 -> Sum/2
  Sum/1 -> Saturation/1
  Saturation/1 -> Math Function/1
  Math Function/1 -> Gain/1
  Gain/1 -> Transfer Fcn/1
  Transfer Fcn/1 -> Sum1/1
  Sum1/1 -> Vusv/1
  Constant1/1 -> Sum1/2

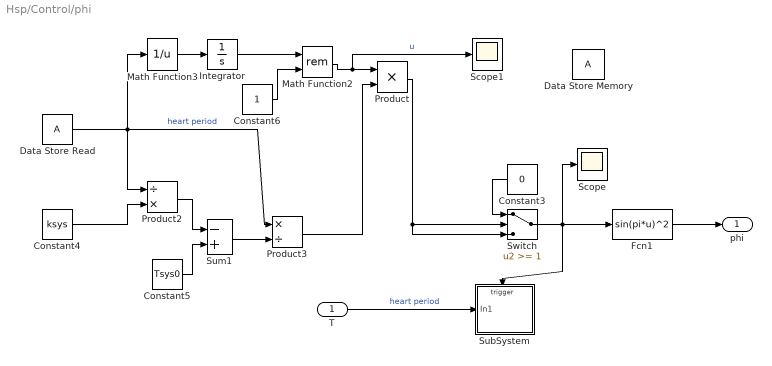
== system Hsp/Control/phi ==
  T : Inport
  Constant3 : Constant  Value=0
  Constant4 : Constant  Value=ksys
  Constant5 : Constant  Value=Tsys0
  Constant6 : Constant
  Data Store Memory : DataStoreMemory  InitialValue=initx(7)  ShowAdditionalParam=off
  Data Store Read : DataStoreRead  SampleTime=0
  Fcn1 : Fcn  Expr=sin(pi*u)^2
  Integrator : Integrator
  Math Function2 : Math  Operator=rem  SaturateOnIntegerOverflow=on
  Math Function3 : Math  Operator=reciprocal  SaturateOnIntegerOverflow=on
  Product : Product  SaturateOnIntegerOverflow=on  RndMeth=Zero  InputSameDT=on  OutDataTypeStr=Inherit: Same as first input
  Product2 : Product  Inputs=/*  SaturateOnIntegerOverflow=on  RndMeth=Zero  InputSameDT=on  OutDataTypeStr=Inherit: Same as first input
  Product3 : Product  Inputs=*/  SaturateOnIntegerOverflow=on  RndMeth=Zero  InputSameDT=on  OutDataTypeStr=Inherit: Same as first input
  Scope : Scope
  Scope1 : Scope
  SubSystem : Subsystem  TreatAsAtomicUnit=on
  Sum1 : Sum  Inputs=-+  SaturateOnIntegerOverflow=on  InputSameDT=on  OutDataTypeStr=Inherit: Same as first input
  Switch : Switch  Threshold=1  SaturateOnIntegerOverflow=on  InputSameDT=on
  phi : Outport
  wires:
  Product3/1 -> Product/2
  Sum1/1 -> Product3/2
  Constant5/1 -> Sum1/2
  Product2/1 -> Sum1/1
  Constant4/1 -> Product2/2
  Constant3/1 -> Switch/1
  Product/1 -> Switch/2, Switch/3
  Fcn1/1 -> phi/1
  T/1 -> SubSystem/1(In1)  "heart period"
  Switch/1 -> Fcn1/1, SubSystem/Trigger, Scope/1
  Data Store Read/1 -> Product3/1, Product2/1, Math Function3/1  "heart period"
  Constant6/1 -> Math Function2/2
  Math Function2/1 -> Product/1, Scope1/1  "u"
  Math Function3/1 -> Integrator/1
  Integrator/1 -> Math Function2/1

== system Hsp/Left Heart/Pmaxlv--Psa ---------------------- Rlv ==
  Pmax : Inport
  P : Inport  Port=2
  Gain : Gain  Gain=KRlv  SaturateOnIntegerOverflow=on  OutDataTypeStr=Inherit: Same as input  ParamDataTypeStr=Inherit: Same as input
  Product : Product  Inputs=/*  SaturateOnIntegerOverflow=on  RndMeth=Zero  InputSameDT=on  OutDataTypeStr=Inherit: Same as first input
  Saturation : Saturate  UpperLimit=inf  LowerLimit=0.01
  Flow : Outport
  wires:
  Pmax/1 -> Gain/1
  Gain/1 -> Saturation/1
  P/1 -> Product/2
  Saturation/1 -> Product/1
  Product/1 -> Flow/1

== system Hsp/Left Heart/SubSystem ==
  _ : Inport
  + : Inport  Port=2
  Saturation : Saturate  UpperLimit=10000  LowerLimit=0
  Sum : Sum  Inputs=|-+  SaturateOnIntegerOverflow=on  InputSameDT=on  OutDataTypeStr=Inherit: Same as first input
  Out : Outport
  wires:
  _/1 -> Sum/1
  +/1 -> Sum/2
  Sum/1 -> Saturation/1
  Saturation/1 -> Out/1

== system Hsp/Left Heart/SubSystem1 ==
  _ : Inport
  + : Inport  Port=2
  Saturation : Saturate  UpperLimit=10000  LowerLimit=0
  Sum : Sum  Inputs=|-+  SaturateOnIntegerOverflow=on  InputSameDT=on  OutDataTypeStr=Inherit: Same as first input
  Out : Outport
  wires:
  Saturation/1 -> Out/1
  Sum/1 -> Saturation/1
  +/1 -> Sum/2
  _/1 -> Sum/1

== system Hsp/Pulmonary/SubSystem ==
  _ : Inport
  + : Inport  Port=2
  Saturation : Saturate  UpperLimit=10000  LowerLimit=0
  Sum : Sum  Inputs=|-+  SaturateOnIntegerOverflow=on  InputSameDT=on  OutDataTypeStr=Inherit: Same as first input
  Out : Outport
  wires:
  _/1 -> Sum/1
  +/1 -> Sum/2
  Sum/1 -> Saturation/1
  Saturation/1 -> Out/1

== system Hsp/Pulmonary/SubSystem1 ==
  _ : Inport
  + : Inport  Port=2
  Saturation : Saturate  UpperLimit=10000  LowerLimit=0
  Sum : Sum  Inputs=|-+  SaturateOnIntegerOverflow=on  InputSameDT=on  OutDataTypeStr=Inherit: Same as first input
  Out : Outport
  wires:
  _/1 -> Sum/1
  +/1 -> Sum/2
  Sum/1 -> Saturation/1
  Saturation/1 -> Out/1

== system Hsp/Pulmonary/SubSystem2 ==
  _ : Inport
  + : Inport  Port=2
  Saturation : Saturate  UpperLimit=10000  LowerLimit=0
  Sum : Sum  Inputs=|-+  SaturateOnIntegerOverflow=on  InputSameDT=on  OutDataTypeStr=Inherit: Same as first input
  Out : Outport
  wires:
  Saturation/1 -> Out/1
  Sum/1 -> Saturation/1
  +/1 -> Sum/2
  _/1 -> Sum/1

== system Hsp/Right Heart/Pmaxrv--Ppa ---------------------- Rrv ==
  Pmax : Inport
  P : Inport  Port=2
  Gain : Gain  Gain=KRrv  SaturateOnIntegerOverflow=on  OutDataTypeStr=Inherit: Same as input  ParamDataTypeStr=Inherit: Same as input
  Product : Product  Inputs=/*  SaturateOnIntegerOverflow=on  RndMeth=Zero  InputSameDT=on  OutDataTypeStr=Inherit: Same as first input
  Saturation : Saturate  UpperLimit=inf  LowerLimit=0.01
  Flow : Outport
  wires:
  Pmax/1 -> Gain/1
  Gain/1 -> Saturation/1
  P/1 -> Product/2
  Saturation/1 -> Product/1
  Product/1 -> Flow/1

== system Hsp/Right Heart/SubSystem ==
  _ : Inport
  + : Inport  Port=2
  Saturation : Saturate  UpperLimit=10000  LowerLimit=0
  Sum : Sum  Inputs=|-+  SaturateOnIntegerOverflow=on  InputSameDT=on  OutDataTypeStr=Inherit: Same as first input
  Out : Outport
  wires:
  _/1 -> Sum/1
  +/1 -> Sum/2
  Sum/1 -> Saturation/1
  Saturation/1 -> Out/1

== system Hsp/Right Heart/SubSystem1 ==
  _ : Inport
  + : Inport  Port=2
  Saturation : Saturate  UpperLimit=10000  LowerLimit=0
  Sum : Sum  Inputs=|-+  SaturateOnIntegerOverflow=on  InputSameDT=on  OutDataTypeStr=Inherit: Same as first input
  Out : Outport
  wires:
  Saturation/1 -> Out/1
  Sum/1 -> Saturation/1
  +/1 -> Sum/2
  _/1 -> Sum/1

== system Hsp/Systemic/Bleed ==
  Clock : Clock
  Constant : Constant  Value=0
  Ramp : simulink/Sources/Ramp  slope=rate  start=tstart  InitialOutput=0
  Saturation : Saturate  UpperLimit=ulimit  LowerLimit=0
  Switch : Switch  Threshold=tstart  SaturateOnIntegerOverflow=on  InputSameDT=on
  Blood Loss : Outport
  wires:
  Clock/1 -> Switch/2
  Constant/1 -> Switch/3
  Ramp/1 -> Switch/1
  Switch/1 -> Saturation/1
  Saturation/1 -> Blood Loss/1

== system Hsp/Systemic/SubSystem ==
  _ : Inport
  + : Inport  Port=2
  Saturation : Saturate  UpperLimit=10000  LowerLimit=0
  Sum : Sum  Inputs=|-+  SaturateOnIntegerOverflow=on  InputSameDT=on  OutDataTypeStr=Inherit: Same as first input
  Out : Outport
  wires:
  _/1 -> Sum/1
  +/1 -> Sum/2
  Sum/1 -> Saturation/1
  Saturation/1 -> Out/1

== system Hsp/Systemic/SubSystem1 ==
  + : Inport
  _ : Inport  Port=2
  Saturation : Saturate  UpperLimit=10000  LowerLimit=0
  Sum : Sum  Inputs=|+-  SaturateOnIntegerOverflow=on  InputSameDT=on  OutDataTypeStr=Inherit: Same as first input
  Out : Outport
  wires:
  Saturation/1 -> Out/1
  Sum/1 -> Saturation/1
  _/1 -> Sum/2
  +/1 -> Sum/1

== system Hsp/Systemic/SubSystem2 ==
  _1 : Inport
  _2 : Inport  Port=2
  + : Inport  Port=3
  Saturation : Saturate  UpperLimit=10000  LowerLimit=0
  Sum : Sum  Inputs=|--+  SaturateOnIntegerOverflow=on  InputSameDT=on  OutDataTypeStr=Inherit: Same as first input
  Out : Outport
  wires:
  Saturation/1 -> Out/1
  Sum/1 -> Saturation/1
  _1/1 -> Sum/1
  +/1 -> Sum/3
  _2/1 -> Sum/2

== system Hsp/Systemic/SubSystem3 ==
  + : Inport
  _ : Inport  Port=2
  Saturation : Saturate  UpperLimit=10000  LowerLimit=0
  Sum : Sum  Inputs=|+-  SaturateOnIntegerOverflow=on  InputSameDT=on  OutDataTypeStr=Inherit: Same as first input
  Out : Outport
  wires:
  +/1 -> Sum/1
  _/1 -> Sum/2
  Sum/1 -> Saturation/1
  Saturation/1 -> Out/1

== system Hsp/Control/Left Ventricle/SubSystem1 ==
  _ : Inport
  + : Inport  Port=2
  Saturation : Saturate  UpperLimit=10000  LowerLimit=0
  Sum : Sum  Inputs=|-+  SaturateOnIntegerOverflow=on  InputSameDT=on  OutDataTypeStr=Inherit: Same as first input
  Out : Outport
  wires:
  _/1 -> Sum/1
  +/1 -> Sum/2
  Sum/1 -> Saturation/1
  Saturation/1 -> Out/1

== system Hsp/Control/Right Ventricle/SubSystem1 ==
  _ : Inport
  + : Inport  Port=2
  Saturation : Saturate  UpperLimit=10000  LowerLimit=0
  Sum : Sum  Inputs=|-+  SaturateOnIntegerOverflow=on  InputSameDT=on  OutDataTypeStr=Inherit: Same as first input
  Out : Outport
  wires:
  Saturation/1 -> Out/1
  Sum/1 -> Saturation/1
  +/1 -> Sum/2
  _/1 -> Sum/1

== system Hsp/Control/phi/SubSystem ==
  In1 : Inport
  Trigger : TriggerPort  VariantControl=(inherit)
  Data Store Write : DataStoreWrite
  Scope : Scope
  wires:
  In1/1 -> Data Store Write/1, Scope/1
